simulink model "STEP5"  (R2020b)
settings: Solver=ode5  StartTime=0.0  StopTime=10000  FixedStep=.0001  RelTol=1e-3  AbsTol=1e-6
libraries: simulink x1
settings Model: FPTRunName=Active  ExtModeTrigMode=oneshot  ExtModeArmWhenConnect=off  ExtModeAutoUpdateStatusClock=off  Creator=The MathWorks, Inc.  LastModifiedBy=Fong
settings SolverCC: AutoScaleAbsTol=off
settings DataIOCC: SaveFormat=Array  SaveOutput=off  SaveTime=off  ReturnWorkspaceOutputs=off
settings OptimizationCC: BooleanDataType=off  ExpressionDepthLimit=2147483647  InitFltsAndDblsToZero=on  EfficientMapNaN2IntZero=off  LifeSpan=inf  BufferReusableBoundary=off
settings DebuggingCC: SaveWithParameterizedLinksMsg=none  UnderspecifiedInitializationDetection=Classic  MergeDetectMultiDrivingBlocksExec=none  SignalResolutionControl=TryResolveAllWithWarning  MultiTaskDSMMsg=warning  MultiTaskCondExecSysMsg=none  IntegerOverflowMsg=none  FcnCallInpInsideContextMsg=warning  StateNameClashWarn=warning  SFUnexpectedBacktrackingDiag=warning  SFNoUnconditionalDefaultTransitionDiag=warning  SFExecutionAtInitializationDiag=none  IntegerSaturationMsg=none  ArithmeticOperatorsInVariantConditions=warning
settings HardwareCC: ProdBitPerPointer=32  ProdBitPerSizeT=32  ProdBitPerPtrDiffT=32  ProdLargestAtomicFloat=None  ProdIntDivRoundTo=Undefined  ProdEndianess=Unspecified  ProdWordSize=32  ProdHWDeviceType=32-bit Generic  TargetUnknown=on
settings ModelReferenceCC: PropagateSignalLabelsOutOfModel=off
settings SFSimCC: SimUseLocalCustomCode=off  SimParseCustomCode=off  CustomCodeUndefinedFunction=UseInterfaceOnly
settings RTWCC: TemplateMakefile=grt_vc.tmf  RTWUseLocalCustomCode=off
settings CodeAppCC: StateflowObjectComments=on
settings GRTTargetCC: TargetFcnLib=ansi_tfl_tmw.mat  TargetLangStandard=C89/C90 (ANSI)  CombineOutputUpdateFcns=off  GRTInterface=on
settings ConfigComp: CovMetricSettings=dcmtr  CovSaveCumulativeToWorkspaceVar=on  CovSaveSingleToWorkspaceVar=on  CovExternalEMLEnable=off  CovSFcnEnable=off

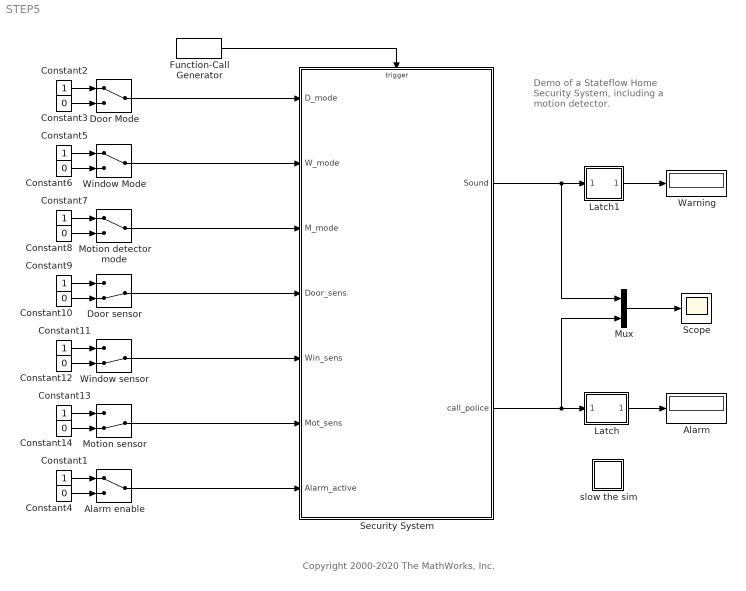
== system STEP5 ==
  note: Demo of a Stateflow
      | Home Security System,
      | including a motion
      | detector.
  note: Copyright 2000-2020 The MathWorks, Inc.
  Alarm : Display
  Alarm enable : ManualSwitch
  Constant{1..2,5,7,9,11,13} (7 alike) : Constant  OutDataTypeStr=boolean
  Constant{3..4,6,8,10,12,14} (7 alike) : Constant  Value=0  OutDataTypeStr=boolean
  Door Mode : ManualSwitch
  Door sensor : ManualSwitch  CurrentSetting=0
  Function-Call Generator : simulink/Ports & Subsystems/Function-Call Generator  sample_time=.05  numberOfIterations=1  DisallowWideOutput=off
  Latch : Subsystem
      mask Display: disp('Hold')
  Latch1 : Subsystem
      mask Display: disp('Hold')
  Motion detector mode : ManualSwitch
  Motion sensor : ManualSwitch  CurrentSetting=0
  Mux : Mux  Inputs=2
  Scope : Scope
  Security System : Stateflow chart  TreatAsAtomicUnit=on
  Warning : Display
  Window Mode : ManualSwitch
  Window sensor : ManualSwitch  CurrentSetting=0
  slow the sim : Subsystem
  wires:
  Latch/1(Trigger) -> Alarm/1
  Door Mode/1 -> Security System/1(D_mode)
  Window Mode/1 -> Security System/2(W_mode)
  Motion detector mode/1 -> Security System/3(M_mode)
  Alarm enable/1 -> Security System/7(Alarm_active)
  Motion sensor/1 -> Security System/6(Mot_sens)
  Window sensor/1 -> Security System/5(Win_sens)
  Door sensor/1 -> Security System/4(Door_sens)
  Function-Call Generator/1 -> Security System/Trigger
  Latch1/1(Trigger) -> Warning/1
  Security System/1(Sound) -> Latch1/1(Reset), Mux/1
  Security System/2(call_police) -> Latch/1(Reset), Mux/2
  Mux/1 -> Scope/1
  Constant4/1 -> Alarm enable/2
  Constant1/1 -> Alarm enable/1
  Constant3/1 -> Door Mode/2
  Constant2/1 -> Door Mode/1
  Constant6/1 -> Window Mode/2
  Constant5/1 -> Window Mode/1
  Constant8/1 -> Motion detector mode/2
  Constant7/1 -> Motion detector mode/1
  Constant10/1 -> Door sensor/2
  Constant12/1 -> Window sensor/2
  Constant11/1 -> Window sensor/1
  Constant14/1 -> Motion sensor/2
  Constant13/1 -> Motion sensor/1
  Constant9/1 -> Door sensor/1

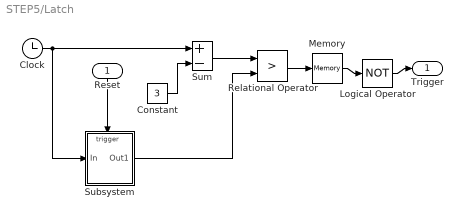
== system STEP5/Latch ==
  Reset : Inport
  Clock : Clock
  Constant : Constant  Value=3
  Logical Operator : Logic  Operator=NOT  Inputs=1
  Memory : Memory  InitialCondition=1
  Relational Operator : RelationalOperator  Operator=>  RndMeth=Nearest  InputSameDT=on
  Subsystem : Subsystem
  Sum : Sum  Inputs=+-  InputSameDT=on  SaturateOnIntegerOverflow=on  OutDataTypeStr=Inherit: Same as first input
  Trigger : Outport  InitialOutput=0  VectorParamsAs1DForOutWhenUnconnected=off
  wires:
  Clock/1 -> Sum/1, Subsystem/1(In)
  Reset/1 -> Subsystem/Trigger
  Constant/1 -> Sum/2
  Sum/1 -> Relational Operator/1
  Subsystem/1(Out1) -> Relational Operator/2
  Relational Operator/1 -> Memory/1
  Memory/1 -> Logical Operator/1
  Logical Operator/1 -> Trigger/1

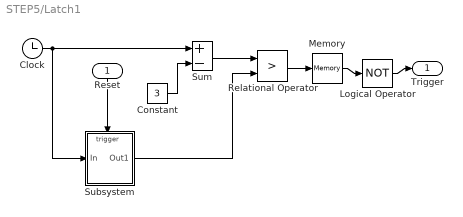
== system STEP5/Latch1 ==
  Reset : Inport
  Clock : Clock
  Constant : Constant  Value=3
  Logical Operator : Logic  Operator=NOT  Inputs=1
  Memory : Memory  InitialCondition=1
  Relational Operator : RelationalOperator  Operator=>  RndMeth=Nearest  InputSameDT=on
  Subsystem : Subsystem
  Sum : Sum  Inputs=+-  InputSameDT=on  SaturateOnIntegerOverflow=on  OutDataTypeStr=Inherit: Same as first input
  Trigger : Outport  InitialOutput=0  VectorParamsAs1DForOutWhenUnconnected=off
  wires:
  Logical Operator/1 -> Trigger/1
  Memory/1 -> Logical Operator/1
  Relational Operator/1 -> Memory/1
  Subsystem/1(Out1) -> Relational Operator/2
  Sum/1 -> Relational Operator/1
  Constant/1 -> Sum/2
  Reset/1 -> Subsystem/Trigger
  Clock/1 -> Subsystem/1(In), Sum/1

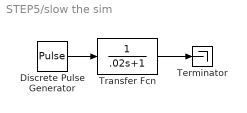
== system STEP5/slow the sim ==
  Discrete Pulse Generator : DiscretePulseGenerator  SampleTime=0.1
  Terminator : Terminator
  Transfer Fcn : TransferFcn  Denominator=[.02 1]
  wires:
  Discrete Pulse Generator/1 -> Transfer Fcn/1
  Transfer Fcn/1 -> Terminator/1

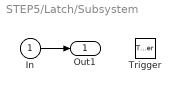
== system STEP5/Latch/Subsystem ==
  In : Inport
  Trigger : TriggerPort  TriggerType=either  VariantControl=Variant
  Out1 : Outport  InitialOutput=-10  VectorParamsAs1DForOutWhenUnconnected=off
  wires:
  In/1 -> Out1/1

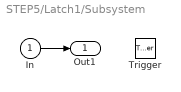
== system STEP5/Latch1/Subsystem ==
  In : Inport
  Trigger : TriggerPort  TriggerType=either  VariantControl=Variant
  Out1 : Outport  InitialOutput=-10  VectorParamsAs1DForOutWhenUnconnected=off
  wires:
  In/1 -> Out1/1

== stateflow chart STEP5/Security System ==
  state The Door and Win states model anti-intrusion sensors at a window and a [group]
    door. When these sensors are active, the corresponding states check the
    value of D_mode and W_mode. If one of these variables is true, the states
    broadcast a local event to the Alarm state.
  state Input from the motion sensor can be sporadic, so a [group]
    debouncing state is used. The debouncing state
    remains active while Mot_sens is true. After a delay
    period, the debouncing state broadcasts a local
    event to the Alert state.
  state Motion [parallel]
    settings: executionOrder=2  description=This state models the modes of a motion detector sensor and implements logic to respond when that sensor is producing a signal.
    state Active
      state Debouncing
      state Idle
      Debouncing -> Debouncing [order 1] : after(1/tSample,sl_call)
          | [in(Alarm.On.Idle)] /{
          | send(Alert,Alarm);}
      Debouncing -> Motion.Active.Idle [order 2] : [~Mot_sens]
      Motion.Active.Idle -> Debouncing : [Mot_sens]
    state Disabled
    (default) -> Motion.Active.Idle
      settings: description=On the first sample call the motion sensor mode is set to active, in the idle substate.
    Motion.Disabled -> Motion.Active.Idle : [M_mode==1]
    Motion.Active -> Motion.Disabled : [M_mode==0]
  state Door [parallel]
    settings: executionOrder=1  description=This state models the modes of a door sensor and implements logic to respond when that sensor is producing a signal.
    state Disabled
    state Active
      Door.Active -> (junction 46) [order 1] : [Door_sens && ...
          |  in(Alarm.On.Idle)]
          | {send(Alert,Alarm);}
    Door.Disabled -> Door.Active : [D_mode==1]
    (default) -> Door.Active
      settings: description=On the first sample call the door mode is set to active.
    Door.Active -> Door.Disabled [order 1] : [D_mode==0]
  state Win [parallel]
    settings: executionOrder=3  description=This state models the modes of a window sensor and implements logic to respond when that sensor is producing a signal.
    state Disabled
    state Active
      Win.Active -> (junction 43) [order 1] : [Win_sens && ...
          | in(Alarm.On.Idle)]
          | {send(Alert,Alarm);}
    Win.Disabled -> Win.Active : [W_mode==1]
    (default) -> Win.Active
      settings: description=On the first sample call the window mode is set to active.
    Win.Active -> Win.Disabled [order 1] : [W_mode==0]
  state Alarm [parallel]
    settings: executionOrder=4
    state On
      state Pending
        entry: Sound;
      state Idle
      (default) -> Alarm.On.Idle
      Alarm.On.Idle -> Pending : Alert
      Pending -> Alarm.On.Idle : after(4/tSample,sl_call)/
          | {call_police;}
    state Off
    (default) -> On
      settings: description=On the first sample call the Alarm is set to active.
    On -> Off : [Alarm_active==0]
    Off -> On : [Alarm_active==1]
  state When an Alert event is [group]
    broadcast to the Alarm state,
    the Pending state becomes
    activate for a delay period.
    If the alarm is not disabled
    during the delay period, the
    police are contacted by the
    output event call_police.
  data: D_mode input boolean; W_mode input boolean; M_mode input boolean; Door_sens input boolean; Win_sens input boolean; Mot_sens input boolean; Alarm_active input boolean; tSample constant double =0.05
  events: Sound output EITHER_EDGE_EVENT; call_police output EITHER_EDGE_EVENT; Alert local EITHER_EDGE_EVENT; sl_call input FUNCTION_CALL_EVENT
